simulink library "thc"  (R2021b)
settings: Solver=VariableStepAuto  StartTime=0.0  StopTime=10.0  RelTol=1e-3
undefined symbols (not defined in the file or in its folder): ATHC_APTCQA_X_C, ATHC_APTCQB_X_C, ATHC_dAy_X_C, ATHC_Qeq_X_kmh, ATHC_VbaseC_X_C, ATHC_VbaseC_Y_W, ATHC_VbaseD_X_C, ATHC_VbaseH_X_C, FALSE, KTHC_ACMaxMinT_sec, KTHC_aDeice_K, KTHC_AGSDefLv_K, KTHC_AGSLv1_K, KTHC_AGSLv2_K, KTHC_AGSLv3_K, KTHC_AGSLv4_K, KTHC_AGSLv5_K, KTHC_AirIntUpdateT_sec, KTHC_APTCOneZoneMax_W, KTHC_APTCQMaxC_W, KTHC_APTCQminC_W, KTHC_APTCQminD_W, KTHC_APTCQminRe1_W, KTHC_APTCQminRe_W, KTHC_APTCQoffT_cnt, KTHC_APTCQonT_cnt, KTHC_APTCRiLeMaxDff_W, KTHC_APTCRiLeMinDff_W, KTHC_BatInTempDef_C, KTHC_bDeice_K, KTHC_CompMaxDeice_rpm, KTHC_CompMinDeice_rpm, KTHC_CompSotxvOp_K, KTHC_CompSotxvOpLow_rpm, KTHC_CompSpdmax_rpm, KTHC_CompSpdmaxBC1_rpm, KTHC_CompSpdmaxBC_rpm, KTHC_CompSpdmid1_rpm, KTHC_CompSpdmid2_rpm, KTHC_CompSpdmid3_rpm, KTHC_CompSpdmid_rpm, KTHC_CompSpdmin_rpm, KTHC_DAPTCQ1_W, KTHC_DAPTCQ2_W, KTHC_DAPTCQ3_W, KTHC_DcChSetTemp_C, KTHC_DehumidityEN_flg, KTHC_DeiceCycTime_K, KTHC_DTambSat1_C, KTHC_DTambSat2_C, KTHC_DTambsat3_C, KTHC_DTambsat4_C, KTHC_DTambSat5_C, KTHC_DTambSat_C, KTHC_DTcabin10_C, KTHC_DTCabin11_C, KTHC_DTcabin12_C, KTHC_DTcabin1_C, KTHC_DTcabin2_C, KTHC_DTcabin3_C ... (+347)
libraries: simulink x80
(part 2 of 8)

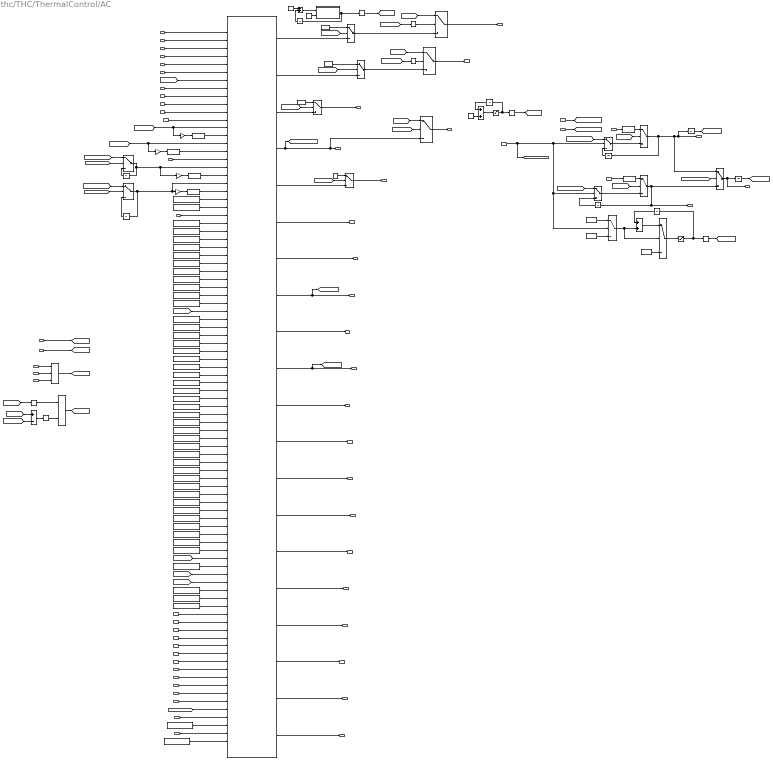
== system thc/THC/ThermalControl/AC ==
  VINP_FCPFrEvtBtnACMaxReq_flg : Inport
  VINP_FCPFrEvtBtnACReq_flg : Inport  Port=2
  VINP_FCPFrEvtBtnAutoReq_flg : Inport  Port=3
  VINP_FCPFrEvtBtnSyncReq_flg : Inport  Port=4
  VINP_Tamb_C : Inport  Port=5
  VINP_Tincar_C : Inport  Port=6
  VINP_sigAirIntenZon1Req_enum : Inport  Port=7
  VINP_sigRecircReq_flg : Inport  Port=8
  VINP_sigFaceReq_flg : Inport  Port=9
  VINP_sigFootReq_flg : Inport  Port=10
  VINP_sigFrostReq_flg : Inport  Port=11
  VINP_sigSetTempZon1Req_C : Inport  Port=12
  VINP_CANMsgValidIVI2_flg : Inport  Port=13
  VINP_sigSetTempZon2Req_C : Inport  Port=14
  VTHC_FDBlowerCmd_pct : Inport  Port=15
  PwrSta : Inport  Port=16
  OFF_AC_MODE : Inport  Port=17
  CabinMode : Inport  Port=18
  T_Foot_L : Inport  Port=19
  T_Foot_R : Inport  Port=20
  T_Foot_Rr : Inport  Port=21
  EEP_ACModeMem : Inport  Port=22
  EEP_Face : Inport  Port=23
  EEP_Foot : Inport  Port=24
  EEP_Frost : Inport  Port=25
  EEP_FaceM : Inport  Port=26
  EEP_FootM : Inport  Port=27
  EEP_CCUSyncSts : Inport  Port=28
  EEP_ACForceOFF : Inport  Port=29
  EEP_sigRecircSt : Inport  Port=30
  EEP_RecAutoFlg : Inport  Port=31
  EEP_AirIntenZone1M : Inport  Port=32
  EEP_fdefog : Inport  Port=33
  EEP_sigSetTempZon1Req : Inport  Port=34
  EEP_sigSetTempZon2Req : Inport  Port=35
  VINP_RemoteAutoReq_flg : Inport  Port=36
  ACSubMode : Inport  Port=37
  Add : Sum
  Add2 : Sum
  Add3 : Sum  Inputs=+-
  Add4 : Sum
  Chart : Stateflow chart  TreatAsAtomicUnit=on
      settings: PortSchema="{\"entries\":[{\"content\":{\"sides\":[{\"content\":{\"connectorIds\":[\"In1\",\"In2\",\"In3\",\"In4\",\"In5\",\"In6\",\"In7\",\"In8\",\"In9\",\"In10\",\"In11\",\"In12\",\"In13\",\"In14\",\"In15\",\"In16\",\"In17\",\"In18\",\"In20\",\"In21\",\"In19\",\"In22\",\"In23\",\"In24\",\"In25\",\"In26\",\"In27\",\"In28\",\"In29\",\"In30\",\"In31\",\"In32\",\"In33\",\"In34\",\"In35\",\"In36\",\"In37\",\"In38\",\"In39\",\"In40\",\"In41\",\"In42\",\"In43\",\"In44\",\"In45\",\"In46\",\"In47\",\"In48\",\"In49\",\"In50\",\"In51\",\"In52\",\"In53\",\"In54\",\"In55\",\"In56\",\"In57\",\"In58\",\"In59\",\"In60\",\"In61\",\"In62\",\"In63\",\"In64\",\"In65\",\"In66\",\"In67\",\"In68\",\"In69\",\"In70\",\"In71\",\"In72\",\"In73\",\"In74\",\"In75\",\"In76\",\"In77\",\"In78\",\"In79\",\"In80\",\"In81\",\"In82\",\"In83\",\"In84\",\"In85\",\"In86\",\"In87\",\"In88\",\"In89\",\"In90\"]},\"type\":\"ConnectorPlacement.EquallySpacedRectSide\",\"uuid\":\"5820fc40-35f0-4b43-a348-a95be02a5108\"},{\"content\":{\"connectorIds\":[\"Out1\",\"Out6\",\"Out2\",\"Out3\",\"Out4\",\"Out5\",\"Out7\",\"Out8\",\"Out9\",\"Out10\",\"Out11\",\"Out12\",\"Out13\",\"Out14\",\"Out15\",\"Out16\",\"Out17\",\"Out18\",\"Out19\",\"Out20\"],\"side\":\"RIGHT\"},\"type\":\"ConnectorPlacement.EquallySpacedRectSide\",\"uuid\":\"36d6613c-bf09-4a00-b7cd-6c94d14300cf\"},{\"content\":{\"connectorIds\":[],\"side\":\"TOP\"},\"type\":\"ConnectorPlacement.EquallySpacedRectSide\",\"uuid\":\"1ae2c247-46e8-45cc-9ea1-ac445f4d9fda\"}]},\"type\":\"ConnectorPlacement.EquallySpacedConnector\",\"uuid\":\"a8684177-dc23-416a-a392-32f98192c4b4\"}],\"packageUris\":[\"http://schema.mathworks.com/mf0/Connector/R2020b\"],\"version\":\"1.0\"}"
  Compare To Constant : simulink/Logic and Bit Operations/Compare To Constant  relop=<  const=5  OutDataTypeStr=boolean
  Compare To Constant2 : simulink/Logic and Bit Operations/Compare To Constant  relop=>=  const=100  OutDataTypeStr=boolean
  Compare To Constant3 : simulink/Logic and Bit Operations/Compare To Constant  relop===  const=3.0  OutDataTypeStr=boolean
  Compare To Constant4 : simulink/Logic and Bit Operations/Compare To Constant  relop=<  const=0  OutDataTypeStr=boolean
  Compare To Constant5 : simulink/Logic and Bit Operations/Compare To Constant  relop=<  const=3.0  OutDataTypeStr=boolean
  Compare To Constant6 : simulink/Logic and Bit Operations/Compare To Constant  relop===  const=2  OutDataTypeStr=boolean
  Compare To Constant7 : simulink/Logic and Bit Operations/Compare To Constant  relop===  const=1  OutDataTypeStr=boolean
  Constant : Constant
  Constant1 : Constant  Value=10
  Constant10 : Constant  Value=KTHC_T2Mmaxamb_C
  Constant11 : Constant  Value=KTHC_T3Mmaxamb_C
  Constant12 : Constant  Value=KTHC_T4Mmaxamb_C
  Constant13 : Constant  Value=KTHC_T3Mminamb_C
  Constant14 : Constant  Value=KTHC_T4Mminamb_C
  Constant15 : Constant  Value=KTHC_T5Mminamb_C
  Constant16 : Constant  Value=KTHC_RecyHold_min
  Constant17 : Constant  Value=KTHC_RecyChange_min
  Constant18 : Constant  Value=KTHC_Tmidlevel_C
  Constant19 : Constant  Value=KTHC_Thilevel1_C
  Constant2 : Constant  Value=FALSE
  Constant20 : Constant  Value=KTHC_Thilevel2_C
  Constant21 : Constant  Value=KTHC_WDZ1Face_flg
  Constant22 : Constant  Value=KTHC_WDZ1Foot_flg
  Constant23 : Constant  Value=KTHC_WDZ1Frost_flg
  Constant24 : Constant  Value=KTHC_WDZ2Face_flg
  Constant25 : Constant  Value=KTHC_WDZ2Foot_flg
  Constant26 : Constant  Value=KTHC_WDZ2Frost_flg
  Constant27 : Constant  Value=KTHC_WDZ3Face_flg
  Constant28 : Constant  Value=KTHC_WDZ3Foot_flg
  Constant29 : Constant  Value=KTHC_WDZ3Frost_flg
  Constant3 : Constant  Value=FALSE
  Constant30 : Constant  Value=KTHC_WDZ4Face_flg
  Constant31 : Constant  Value=KTHC_WDZ4Foot_flg
  Constant32 : Constant  Value=KTHC_WDZ4Frost_flg
  Constant33 : Constant  Value=KTHC_WDZ5Face_flg
  Constant34 : Constant  Value=KTHC_WDZ5Foot_flg
  Constant35 : Constant  Value=KTHC_WDZ5Frost_flg
  Constant36 : Constant  Value=KTHC_WDZ6Face_flg
  Constant37 : Constant  Value=KTHC_WDZ6Foot_flg
  Constant38 : Constant  Value=KTHC_WDZ6Frost_flg
  Constant39 : Constant  Value=KTHC_WDZ7Face_flg
  Constant4 : Constant  Value=ZERO_INT
  Constant40 : Constant  Value=KTHC_WDZ7Foot_flg
  Constant41 : Constant  Value=KTHC_WDZ7Frost_flg
  Constant42 : Constant  Value=KTHC_WDZ8Face_flg
  Constant43 : Constant  Value=KTHC_WDZ8Foot_flg
  Constant44 : Constant  Value=KTHC_WDZ8Frost_flg
  Constant45 : Constant  Value=KTHC_WDZ9Face_flg
  Constant46 : Constant  Value=KTHC_WDZ9Foot_flg
  Constant47 : Constant  Value=KTHC_WDZ9Frost_flg
  Constant48 : Constant  Value=ONE_INT
  Constant49 : Constant  Value=ZERO_INT
  Constant5 : Constant  Value=KTHC_RecyOutterD_enum
  Constant50 : Constant  Value=KTHC_Trecymin_C
  Constant51 : Constant  Value=KTHC_RefreshEN_flg
  Constant52 : Constant  Value=KTHC_FootColdT_C
  Constant53 : Constant  Value=KTHC_FootColdTdelta_C
  Constant54 : Constant  Value=KTHC_ACMaxMinT_sec
  Constant55 : Constant
  Constant56 : Constant  Value=FALSE
  Constant57 : Constant  Value=KTHC_WDZ10Foot_flg
  Constant58 : Constant  Value=KTHC_WDZ10Frost_flg
  Constant6 : Constant  Value=KTHC_WDZ10Face_flg
  Constant7 : Constant  Value=KTHC_WindDirUpdateT_min
  Constant8 : Constant
  Constant9 : Constant  Value=KTHC_AirIntUpdateT_sec
  Data Type Conversion : DataTypeConversion  OutDataTypeStr=single
  Data Type Conversion1 : DataTypeConversion  OutDataTypeStr=single
  Data Type Conversion{2..5} (4 alike) : DataTypeConversion  OutDataTypeStr=uint16
  Gain{,1..3} (4 alike) : Gain  Gain=10
  Logical Operator : Logic  Operator=NXOR  AllPortsSameDT=off  OutDataTypeStr=boolean
  Min : MinMax  Inputs=3
  ModMath2 : Subsystem  mask(Count){}
      mask help: Counter function.
      mask Display:
      | fprintf('ModMath');
      | port_label('output', 1, 'Remainder');
      | port_label('input', 1, 'Dividend');
      | port_label('input', 2, 'Divisor');
  Saturation : Saturate  UpperLimit=100  LowerLimit=0
  Saturation1 : Saturate  UpperLimit=3  LowerLimit=0
  Switch{,1..15} (16 alike) : Switch  Criteria=u2 > Threshold
  Unit Delay : UnitDelay  InitialCondition=26  SampleTime=-1  HasFrameUpgradeWarning=on
  Unit Delay1 : UnitDelay  InitialCondition=26  SampleTime=-1  HasFrameUpgradeWarning=on
  Unit Delay{2..8} (7 alike) : UnitDelay  SampleTime=-1  HasFrameUpgradeWarning=on
  VTHC_CCUACLampSts_flg : Outport
  VTHC_CCUAutoLampSts_flg : Outport  Port=2
  VTHC_CCUACMaxLampSts_flg : Outport  Port=3
  VTHC_CCUSyncLampSts_flg : Outport  Port=4
  VTHC_sigAirIntenZon1St_enum : Outport  Port=5
  VTHC_sigWindDirZon1St_enum : Outport  Port=6
  VTHC_sigRecircSt_flg : Outport  Port=7
  VTHC_sigSetTempZon1St_C : Outport  Port=8
  VTHC_sigSetTempZon2St_C : Outport  Port=9
  WaterFillReq : Outport  Port=10
  PET : Outport  Port=11
  FD_RecyAuto_Cmd : Outport  Port=12
  ACModeMem : Outport  Port=13
  Face : Outport  Port=14
  Foot : Outport  Port=15
  Frost : Outport  Port=16
  FaceM : Outport  Port=17
  FootM : Outport  Port=18
  CCUSyncSts : Outport  Port=19
  ACForceOFF : Outport  Port=20
  RecAutoFlg : Outport  Port=21
  AirIntenZone1M : Outport  Port=22
  fdefog : Outport  Port=23
  VTHC_sigSetTempZon2StM_C : Outport  Port=24
  wires:
  Unit Delay1/1 -> Switch2/3
  Switch11/1 -> Unit Delay/1, Switch/1, Unit Delay3/1, VTHC_sigSetTempZon1St_C/1  "VTHC_sigSetTempZon1St_C"
  [VTHC_CCUSyncSts_flg] -> Switch/2
  VINP_Tamb_C/1 -> Chart/6(Tamb)
  VINP_sigAirIntenZon1Req_enum/1 -> Chart/8(sigAirIntenZon1Req)
  Chart/7(sigRecircSt) -> VTHC_sigRecircSt_flg/1  "VTHC_sigRecircSt_flg"
  Chart/1(CCU_ACLampSts) -> Switch4/3  "VTHC_CCUACLampSts_flg"
  VINP_FCPFrEvtBtnACMaxReq_flg/1 -> Chart/1(FCP_FrEvt_BtnACMaxReq)
  Chart/5(sigWindDirZon1St) -> VTHC_sigWindDirZon1St_enum/1  "VTHC_sigWindDirZon1St_enum"
  VINP_sigFrostReq_flg/1 -> Chart/12(sigFrostReq)
  VINP_sigRecircReq_flg/1 -> Chart/9(sigRecircReq)
  Switch/1 -> VTHC_sigSetTempZon2St_C/1, Unit Delay7/1  "VTHC_sigSetTempZon2St_C"
  VINP_sigFaceReq_flg/1 -> Chart/10(sigFaceReq)
  VINP_sigFootReq_flg/1 -> Chart/11(sigFootReq)
  VINP_FCPFrEvtBtnSyncReq_flg/1 -> Chart/4(FCP_FrEvt_BtnSyncReq)
  VINP_FCPFrEvtBtnACReq_flg/1 -> Chart/2(FCP_FrEvt_BtnACReq)
  VINP_FCPFrEvtBtnAutoReq_flg/1 -> Chart/3(FCP_FrEvt_BtnAutoReq)
  VINP_CANMsgValidIVI2_flg/1 -> [VINP_CANMsgValidIVI2_flg], Switch1/2, Switch9/2, Switch2/2  "VINP_CANMsgValidIVI2_flg"
  Chart/2(CCU_ACMaxLampSts) -> Switch5/3  "VTHC_CCUACMaxLampSts_flg"
  VTHC_FDBlowerCmd_pct/1 -> Chart/5(FD_Blower_Cmd)
  PwrSta/1 -> Chart/17(PwrSta)
  Chart/9(Frost) -> Frost/1
  Chart/8(WaterFillReq) -> [WaterFillReq], WaterFillReq/1
  Add/1 -> ModMath2/1(Dividend)
  Unit Delay4/1 -> Add/2
  Constant/1 -> Add/1
  Constant1/1 -> ModMath2/2(Divisor)
  [WaterFillReq] -> Compare To Constant7/1
  Chart/10(ACForceOFF) -> [ACForceOFF], ACForceOFF/1
  [ACForceOFF] -> Switch4/2
  Switch4/1 -> Switch3/3  "VTHC_CCUACLampSts_flg"
  Constant2/1 -> Switch4/1
  Switch5/1 -> VTHC_CCUACMaxLampSts_flg/1  "VTHC_CCUACMaxLampSts_flg"
  [ACForceOFF] -> Switch5/2
  Constant3/1 -> Switch5/1
  Switch3/1 -> VTHC_CCUACLampSts_flg/1  "VTHC_CCUACLampSts_flg"
  [ACForceOFF] -> Switch6/2
  Constant56/1 -> Switch6/1
  Chart/3(CCU_SyncSts) -> Switch7/3, CCUSyncSts/1, [VTHC_CCUSyncSts_flg]
  [Flash] -> Switch7/1
  [ACForceOFF] -> Switch7/2
  Switch7/1 -> VTHC_CCUSyncLampSts_flg/1  "VTHC_CCUSyncLampSts_flg"
  Constant7/1 -> Chart/22(KTHC_WindDirUpdateT_min)
  Constant8/1 -> Switch8/1
  [ACForceOFF] -> Switch8/2
  Switch8/1 -> VTHC_sigAirIntenZon1St_enum/1  "VTHC_sigAirIntenZon1St_enum"
  Chart/4(sigAirIntenZon1St) -> Switch8/3
  VINP_sigSetTempZon2Req_C/1 -> [VINP_sigSetTempZon2Req_C]
  VINP_sigSetTempZon1Req_C/1 -> [VINP_sigSetTempZon1Req_C]
  [VINP_sigSetTempZon1Req_C] -> Switch1/1
  [VINP_sigSetTempZon2Req_C] -> Switch2/1
  Constant9/1 -> Chart/23(KTHC_AirIntUpdateT_sec)
  OFF_AC_MODE/1 -> Chart/24(OFF_AC_MODE)
  Chart/11(PET) -> PET/1
  Constant10/1 -> Chart/25(KTHC_T2Mmaxamb_C)
  Constant11/1 -> Chart/26(KTHC_T3Mmaxamb_C)
  Constant12/1 -> Chart/27(KTHC_T4Mmaxamb_C)
  Constant13/1 -> Chart/28(KTHC_T3Mminamb_C)
  Constant14/1 -> Chart/29(KTHC_T4Mminamb_C)
  Constant15/1 -> Chart/30(KTHC_T5Mminamb_C)
  Constant16/1 -> Chart/31(KTHC_RecyHold_min)
  Constant17/1 -> Chart/32(KTHC_RecyChange_min)
  Chart/12(FD_RecyAuto_Cmd) -> FD_RecyAuto_Cmd/1
  Constant18/1 -> Chart/33(KTHC_Tmidlevel_C)
  Constant19/1 -> Chart/34(KTHC_Thilevel1_C)
  Constant20/1 -> Chart/35(KTHC_Thilevel2_C)
  Constant21/1 -> Chart/37(KTHC_WDZ1Face_flg)
  Constant23/1 -> Chart/39(KTHC_WDZ1Frost_flg)
  Constant22/1 -> Chart/38(KTHC_WDZ1Foot_flg)
  Constant24/1 -> Chart/40(KTHC_WDZ2Face_flg)
  Constant25/1 -> Chart/41(KTHC_WDZ2Foot_flg)
  Constant26/1 -> Chart/42(KTHC_WDZ2Frost_flg)
  Constant27/1 -> Chart/43(KTHC_WDZ3Face_flg)
  Constant28/1 -> Chart/44(KTHC_WDZ3Foot_flg)
  Constant29/1 -> Chart/45(KTHC_WDZ3Frost_flg)
  Constant30/1 -> Chart/46(KTHC_WDZ4Face_flg)
  Constant31/1 -> Chart/47(KTHC_WDZ4Foot_flg)
  Constant32/1 -> Chart/48(KTHC_WDZ4Frost_flg)
  Constant33/1 -> Chart/49(KTHC_WDZ5Face_flg)
  Constant34/1 -> Chart/50(KTHC_WDZ5Foot_flg)
  Constant35/1 -> Chart/51(KTHC_WDZ5Frost_flg)
  Constant36/1 -> Chart/52(KTHC_WDZ6Face_flg)
  Constant37/1 -> Chart/53(KTHC_WDZ6Foot_flg)
  Constant38/1 -> Chart/54(KTHC_WDZ6Frost_flg)
  Constant39/1 -> Chart/55(KTHC_WDZ7Face_flg)
  Constant40/1 -> Chart/56(KTHC_WDZ7Foot_flg)
  Constant41/1 -> Chart/57(KTHC_WDZ7Frost_flg)
  Constant42/1 -> Chart/58(KTHC_WDZ8Face_flg)
  Constant43/1 -> Chart/59(KTHC_WDZ8Foot_flg)
  Constant44/1 -> Chart/60(KTHC_WDZ8Frost_flg)
  Constant45/1 -> Chart/61(KTHC_WDZ9Face_flg)
  Constant46/1 -> Chart/62(KTHC_WDZ9Foot_flg)
  Constant47/1 -> Chart/63(KTHC_WDZ9Frost_flg)
  Constant49/1 -> Switch9/1
  Constant48/1 -> Switch9/3
  Switch9/1 -> Switch10/2, Add2/2
  Add2/1 -> Switch10/1
  Constant4/1 -> Switch10/3
  Switch10/1 -> Saturation/1
  Unit Delay6/1 -> Add2/1
  Saturation/1 -> Compare To Constant2/1, Unit Delay6/1
  Compare To Constant2/1 -> [ForceAuto]
  [ForceAuto] -> Chart/67(ForceAuto)
  Constant51/1 -> Chart/68(KTHC_RefreshEN_flg)
  T_Foot_L/1 -> Min/1
  T_Foot_R/1 -> Min/2
  T_Foot_Rr/1 -> Min/3
  Min/1 -> [T_Foot_min]
  [T_Foot_min] -> Chart/70(T_Foot_min)
  Constant52/1 -> Chart/71(KTHC_FootColdT_C)
  Constant53/1 -> Chart/72(KTHC_FootColdTdelta_C)
  CabinMode/1 -> [CabinMode]
  [CabinMode] -> Chart/36(CabinMode)
  [CabinMode] -> Compare To Constant3/1
  VINP_Tincar_C/1 -> [Tincar]
  [Tincar] -> Chart/7(Tincar)
  [Tincar] -> Add3/1
  [sigSetTempZon1St] -> Add3/2
  Add3/1 -> Compare To Constant4/1
  Compare To Constant3/1 -> Logical Operator/1
  Compare To Constant4/1 -> Logical Operator/2
  Logical Operator/1 -> [MaxFinish]
  [MaxFinish] -> Chart/69(MaxFinish)
  Constant54/1 -> Chart/73(KTHC_ACMaxMinT_sec)
  EEP_ACModeMem/1 -> Chart/74(EEP_ACModeMem)
  EEP_Face/1 -> Chart/75(EEP_Face)
  EEP_Foot/1 -> Chart/76(EEP_Foot)
  EEP_Frost/1 -> Chart/77(EEP_Frost)
  EEP_FaceM/1 -> Chart/78(EEP_FaceM)
  EEP_FootM/1 -> Chart/79(EEP_FootM)
  EEP_CCUSyncSts/1 -> Chart/80(EEP_CCUSyncSts)
  EEP_ACForceOFF/1 -> Chart/81(EEP_ACForceOFF)
  EEP_sigRecircSt/1 -> Chart/82(EEP_sigRecircSt)
  EEP_RecAutoFlg/1 -> Chart/83(EEP_RecAutoFlg)
  EEP_AirIntenZone1M/1 -> Chart/84(EEP_AirIntenZone1M)
  Chart/13(ACModeMem) -> ACModeMem/1
  Chart/14(FaceM) -> FaceM/1
  Chart/15(FootM) -> FootM/1
  Chart/16(Face) -> Face/1
  Chart/17(Foot) -> Foot/1
  EEP_fdefog/1 -> Chart/85(EEP_fdefog)
  Chart/18(fdefog) -> fdefog/1
  Chart/19(RecAutoFlg) -> RecAutoFlg/1
  Chart/20(AirIntenZone1M) -> AirIntenZone1M/1
  Add4/1 -> Saturation1/1
  Constant55/1 -> Add4/2
  Saturation1/1 -> Unit Delay2/1, Compare To Constant5/1
  Unit Delay2/1 -> Add4/1
  Compare To Constant5/1 -> [fInitial]
  Switch1/1 -> Switch11/3
  [fInitial] -> Switch11/2
  Unit Delay/1 -> Switch1/3
  EEP_sigSetTempZon1Req/1 -> Data Type Conversion/1
  Switch2/1 -> Switch12/3
  [fInitial] -> Switch12/2
  EEP_sigSetTempZon2Req/1 -> Data Type Conversion1/1
  Switch12/1 -> Switch/3, VTHC_sigSetTempZon2StM_C/1, Unit Delay1/1  "VTHC_sigSetTempZon2StM_C"
  [VINP_CANMsgValidIVI2_flg] -> Chart/86(VINP_CANMsgValidIVI2_flg)
  Unit Delay3/1 -> [sigSetTempZon1St]
  Unit Delay7/1 -> [sigSetTempZon2St]
  ModMath2/1(Remainder) -> Unit Delay4/1, Compare To Constant/1
  Data Type Conversion/1 -> Switch11/1
  Data Type Conversion1/1 -> Switch12/1
  Gain/1 -> Data Type Conversion2/1
  Data Type Conversion2/1 -> Chart/14(SetTempZon1St_CMD)
  [sigSetTempZon1St] -> Gain/1, Chart/13(sigSetTempZon1St)
  Data Type Conversion3/1 -> Chart/16(SetTempZon2St_CMD)
  [sigSetTempZon2St] -> Gain1/1, Chart/15(sigSetTempZon2St)
  Gain1/1 -> Data Type Conversion3/1
  VINP_RemoteAutoReq_flg/1 -> Chart/87(VINP_RemoteAutoReq_flg)
  Chart/6(CCU_AutoLampSts) -> Switch6/3  "VTHC_CCUAutoLampSts_flg"
  Switch6/1 -> Switch13/3  "VTHC_CCUAutoLampSts_flg"
  Compare To Constant/1 -> [Flash]
  [Flash] -> Switch3/1
  [Flash] -> Switch13/1
  Switch13/1 -> VTHC_CCUAutoLampSts_flg/1  "VTHC_CCUAutoLampSts_flg"
  [WaterFillReq] -> Compare To Constant6/1
  Compare To Constant6/1 -> Switch13/2
  Compare To Constant7/1 -> Switch3/2
  Constant50/1 -> Chart/88(KTHC_Trecymin_C)
  ACSubMode/1 -> Chart/89(ACSubMode)
  Switch14/1 -> Gain2/1, Chart/18(sigSetTempZon1Req), Unit Delay5/1
  Data Type Conversion4/1 -> Chart/20(sigSetTempZon1Req_CMD)
  Gain2/1 -> Data Type Conversion4/1
  Gain3/1 -> Data Type Conversion5/1
  Data Type Conversion5/1 -> Chart/19(sigSetTempZon2Req_CMD)
  Constant5/1 -> Chart/90(KTHC_RecyOutterD_enum)
  [VINP_sigSetTempZon1Req_C] -> Switch14/1
  Unit Delay5/1 -> Switch14/3
  [VINP_CANMsgValidIVI2_flg] -> Switch14/2
  Switch15/1 -> Chart/21(sigSetTempZon2Req), Gain3/1, Unit Delay8/1
  Unit Delay8/1 -> Switch15/3
  [VINP_sigSetTempZon2Req_C] -> Switch15/1
  [VINP_CANMsgValidIVI2_flg] -> Switch15/2
  Constant6/1 -> Chart/64(KTHC_WDZ10Face_flg)
  Constant57/1 -> Chart/65(KTHC_WDZ10Foot_flg)
  Constant58/1 -> Chart/66(KTHC_WDZ10Frost_flg)
